simulink model "third"  (R2022b)
settings: Solver=VariableStepAuto  StartTime=0.0  StopTime=10.0  RelTol=1e-3
settings Model: Creator=Vikhyath  LastModifiedBy=Vikhyath

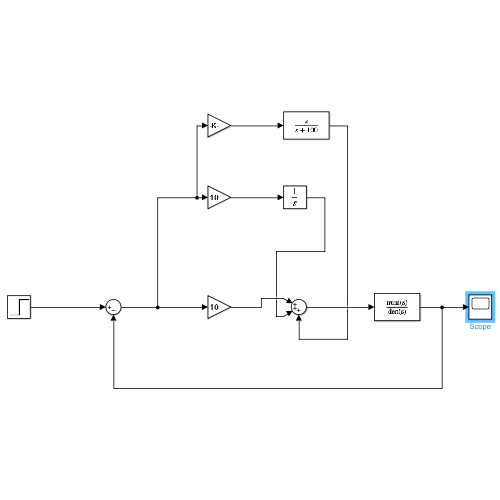
[thumbnail: Simulink's stored preview of the top-level diagram]
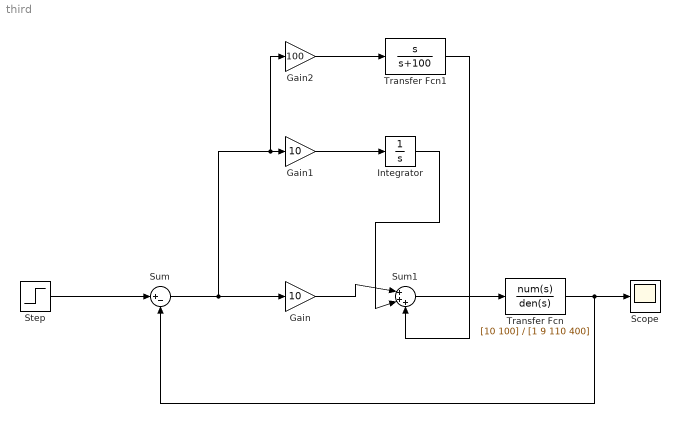
== system third ==
  Gain : Gain  Gain=10
  Gain1 : Gain  Gain=10
  Gain2 : Gain  Gain=100
  Integrator : Integrator
  Scope : Scope
  Step : Step  Time=0  SampleTime=0
  Sum : Sum  Inputs=|+-
  Sum1 : Sum  Inputs=|+++
  Transfer Fcn : TransferFcn  Numerator=[10 100]  Denominator=[1 9 110 400]
  Transfer Fcn1 : TransferFcn  Numerator=[1 0]  Denominator=[1 100]
  wires:
  Sum/1 -> Gain2/1, Gain1/1, Gain/1
  Step/1 -> Sum/1
  Gain1/1 -> Integrator/1
  Gain/1 -> Sum1/1
  Integrator/1 -> Sum1/2
  Sum1/1 -> Transfer Fcn/1
  Transfer Fcn/1 -> Sum/2, Scope/1
  Gain2/1 -> Transfer Fcn1/1
  Transfer Fcn1/1 -> Sum1/3
